simulink model "vehicle_steering_fixed_datatype"  (R2022a)
settings: Solver=VariableStepAuto  StartTime=0.0  StopTime=10  RelTol=1e-3
model workspace (MATLAB code in the model file):
  | bits = 16;
  | a = 0.5;
  | b = 1;
  | gamma = a/b;
  | A = [0, 1; 0, 0];
  | B = [gamma; 1];
  | C = [1, 0];
  | D = 0;
  | 
  | k1 = sfi(1, bits);
  | k2 = sfi(1.6, bits);
  | K = [k1, k2];
  | kr = sfi(1, bits);
  | w_c = sqrt(k1);
  | zi = (k2 + gamma*w_c^2)/(2*w_c);
  | 
  | % w_c = 1;
  | % zi = 0.5;
  | % k1 = w_c^2;
  | % k2 = 2*zi*w_c - gamma*w_c^2;
  | % K = [k1, k2];
settings Model: Creator=ba13  LastModifiedBy=ba13
settings DataIOCC: Refine=20

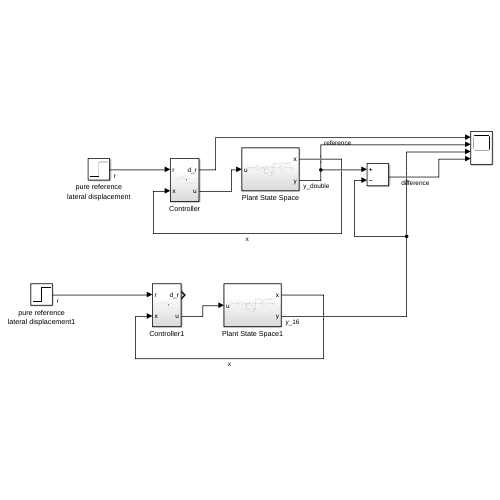
[thumbnail: Simulink's stored preview of the top-level diagram]
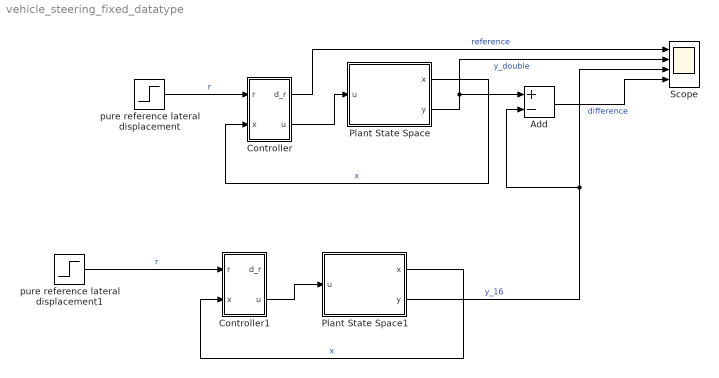
== system vehicle_steering_fixed_datatype ==
  Add : Sum  Inputs=+-
  Controller : Subsystem
  Controller1 : Subsystem
  Plant State Space : Subsystem
  Plant State Space1 : Subsystem
  Scope : Scope  NumInputPorts=4
  pure reference lateral displacement : Step  SampleTime=0
  pure reference lateral displacement1 : Step  SampleTime=0
  wires:
  Plant State Space/1(x) -> Controller/2(x)  "x"
  pure reference lateral displacement/1 -> Controller/1(r)  "r"
  Controller/2(u) -> Plant State Space/1(u)
  Controller/1(d_r) -> Scope/1  "reference"
  Plant State Space1/1(x) -> Controller1/2(x)  "x"
  Plant State Space1/2(y) -> Add/2, Scope/3  "y_16"
  Controller1/2(u) -> Plant State Space1/1(u)
  pure reference lateral displacement1/1 -> Controller1/1(r)  "r"
  Plant State Space/2(y) -> Add/1, Scope/2  "y_double"
  Add/1 -> Scope/4  "difference"

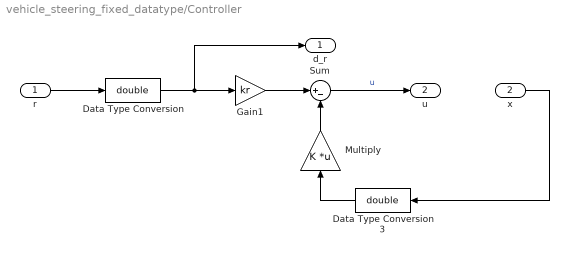
== system vehicle_steering_fixed_datatype/Controller ==
  r : Inport
  x : Inport  Port=2
  Data Type Conversion : DataTypeConversion  OutMin=[-5]  OutMax=[5]  OutDataTypeStr=double  SaturateOnIntegerOverflow=off  RndMeth=Floor
  Data Type Conversion3 : DataTypeConversion  OutMin=[-5]  OutMax=[5]  OutDataTypeStr=double  SaturateOnIntegerOverflow=off  RndMeth=Floor
  Gain1 : Gain  Gain=kr
  Multiply : Gain  Gain=K  Multiplication=Matrix(K*u)
  Sum : Sum  Inputs=|+-
  d_r : Outport
  u : Outport  Port=2
  wires:
  r/1 -> Data Type Conversion/1
  Gain1/1 -> Sum/1
  Multiply/1 -> Sum/2
  Sum/1 -> u/1  "u"
  Data Type Conversion3/1 -> Multiply/1
  Data Type Conversion/1 -> d_r/1, Gain1/1
  x/1 -> Data Type Conversion3/1

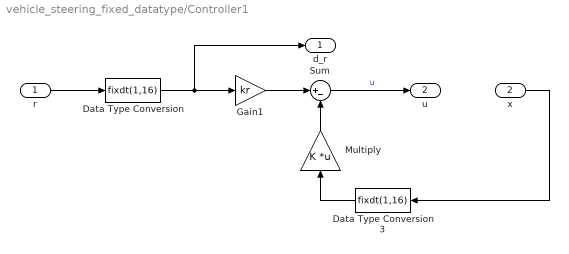
== system vehicle_steering_fixed_datatype/Controller1 ==
  r : Inport
  x : Inport  Port=2
  Data Type Conversion : DataTypeConversion  OutMin=[-5]  OutMax=[5]  OutDataTypeStr=fixdt(1,16)  SaturateOnIntegerOverflow=off  RndMeth=Floor
  Data Type Conversion3 : DataTypeConversion  OutMin=[-5]  OutMax=[5]  OutDataTypeStr=fixdt(1,16)  SaturateOnIntegerOverflow=off  RndMeth=Floor
  Gain1 : Gain  Gain=kr
  Multiply : Gain  Gain=K  Multiplication=Matrix(K*u)
  Sum : Sum  Inputs=|+-
  d_r : Outport
  u : Outport  Port=2
  wires:
  r/1 -> Data Type Conversion/1
  Gain1/1 -> Sum/1
  Multiply/1 -> Sum/2
  Sum/1 -> u/1  "u"
  Data Type Conversion3/1 -> Multiply/1
  Data Type Conversion/1 -> d_r/1, Gain1/1
  x/1 -> Data Type Conversion3/1

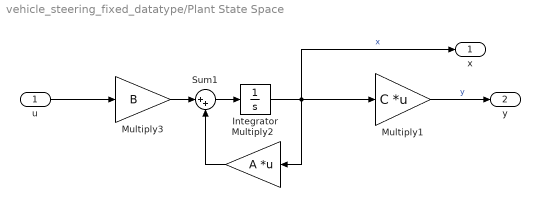
== system vehicle_steering_fixed_datatype/Plant State Space ==
  u : Inport
  Integrator : Integrator
  Multiply1 : Gain  Gain=C  Multiplication=Matrix(K*u)
  Multiply2 : Gain  Gain=A  Multiplication=Matrix(K*u)
  Multiply3 : Gain  Gain=B
  Sum1 : Sum  Inputs=|++
  x : Outport
  y : Outport  Port=2
  wires:
  Multiply2/1 -> Sum1/2
  Sum1/1 -> Integrator/1
  Integrator/1 -> Multiply1/1, x/1, Multiply2/1  "x"
  Multiply3/1 -> Sum1/1
  Multiply1/1 -> y/1  "y"
  u/1 -> Multiply3/1

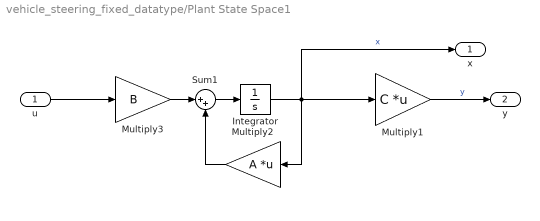
== system vehicle_steering_fixed_datatype/Plant State Space1 ==
  u : Inport
  Integrator : Integrator
  Multiply1 : Gain  Gain=C  Multiplication=Matrix(K*u)
  Multiply2 : Gain  Gain=A  Multiplication=Matrix(K*u)
  Multiply3 : Gain  Gain=B
  Sum1 : Sum  Inputs=|++
  x : Outport
  y : Outport  Port=2
  wires:
  Multiply2/1 -> Sum1/2
  Sum1/1 -> Integrator/1
  Integrator/1 -> Multiply1/1, x/1, Multiply2/1  "x"
  Multiply3/1 -> Sum1/1
  Multiply1/1 -> y/1  "y"
  u/1 -> Multiply3/1
